simulink model "sat_sim"  (R2023b)
settings: Solver=VariableStepAuto  StartTime=0.0  StopTime=100000  RelTol=1e-3
values from neighbouring files (symbols this model uses):
  Dx = 1.0    (= 1)    [satellite.m]
  Dy = 2.0    (= 2)    [satellite.m]
  Dz = 1.0    (= 1)    [satellite.m]
  Iwx = 2    [satellite.m]
  Iwy = 2    [satellite.m]
  Iwz = 2    [satellite.m]
  Ix = 6.916894    [satellite.m]
  Iy = 6.684942    [satellite.m]
  Iz = 4.915737    [satellite.m]
  sx = (Iy-Iz)/Ix    (= 0.255780267849)    [satellite.m]
  sy = (Ix-Iz)/Iy    (= 0.299352933803)    [satellite.m]
  sz = abs(Iy-Ix)/Iz    [satellite.m]
  w0 = v/(RE+h)    (= 0.00108023189236)    [satellite.m]
undefined symbols (not defined in the file or in its folder): c0, c1, c2, c3, c4, c5

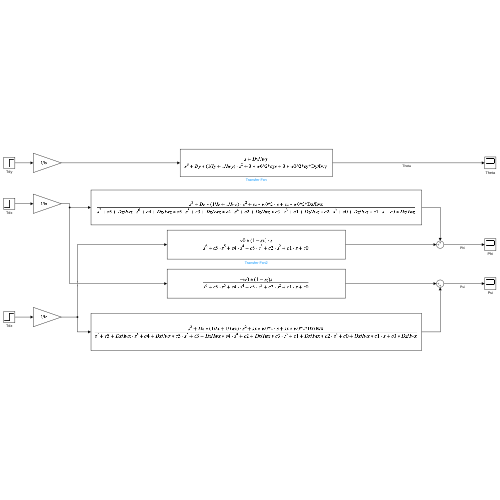
[thumbnail: Simulink's stored preview of the top-level diagram]
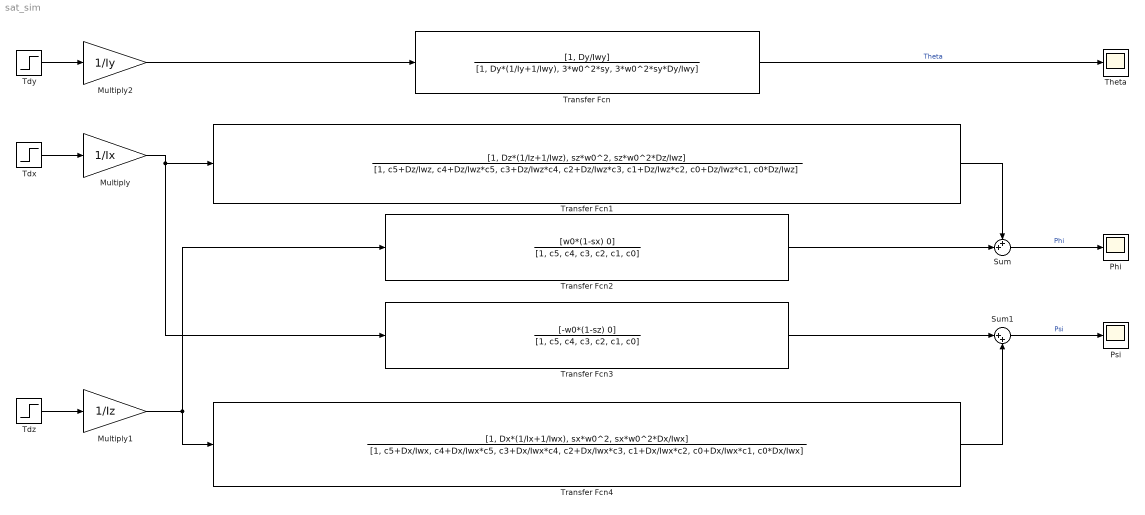
== system sat_sim ==
  Multiply : Gain  Gain=1/Ix
  Multiply1 : Gain  Gain=1/Iz
  Multiply2 : Gain  Gain=1/Iy
  Phi : Scope
  Psi : Scope
  Sum : Sum  Inputs=++|
  Sum1 : Sum  Inputs=|++
  Tdx : Step  SampleTime=0
  Tdy : Step  SampleTime=0
  Tdz : Step  SampleTime=0
  Theta : Scope
  Transfer Fcn : TransferFcn  Numerator=[1, Dy/Iwy]  Denominator=[1, Dy*(1/Iy+1/Iwy), 3*w0^2*sy, 3*w0^2*sy*Dy/Iwy]
  Transfer Fcn1 : TransferFcn  Numerator=[1, Dz*(1/Iz+1/Iwz), sz*w0^2, sz*w0^2*Dz/Iwz]  Denominator=[1, c5+Dz/Iwz, c4+Dz/Iwz*c5, c3+Dz/Iwz*c4, c2+Dz/Iwz*c3, c1+Dz/Iwz*c2, c0+Dz/Iwz*c1, c0*Dz/Iwz]
  Transfer Fcn2 : TransferFcn  Numerator=[w0*(1-sx) 0]  Denominator=[1, c5, c4, c3, c2, c1, c0]
  Transfer Fcn3 : TransferFcn  Numerator=[-w0*(1-sz) 0]  Denominator=[1, c5, c4, c3, c2, c1, c0]
  Transfer Fcn4 : TransferFcn  Numerator=[1, Dx*(1/Ix+1/Iwx), sx*w0^2, sx*w0^2*Dx/Iwx]  Denominator=[1, c5+Dx/Iwx, c4+Dx/Iwx*c5, c3+Dx/Iwx*c4, c2+Dx/Iwx*c3, c1+Dx/Iwx*c2, c0+Dx/Iwx*c1, c0*Dx/Iwx]
  wires:
  Tdy/1 -> Multiply2/1
  Transfer Fcn/1 -> Theta/1  "Theta"
  Tdx/1 -> Multiply/1
  Multiply1/1 -> Transfer Fcn2/1, Transfer Fcn4/1
  Tdz/1 -> Multiply1/1
  Multiply/1 -> Transfer Fcn3/1, Transfer Fcn1/1
  Transfer Fcn1/1 -> Sum/1
  Transfer Fcn2/1 -> Sum/2
  Sum/1 -> Phi/1  "Phi"
  Transfer Fcn3/1 -> Sum1/1
  Transfer Fcn4/1 -> Sum1/2
  Sum1/1 -> Psi/1  "Psi"
  Multiply2/1 -> Transfer Fcn/1
